simulink model "bh_test_generic_MLFB_model"  (R2021a)
settings: Solver=ode4  StartTime=0.0  StopTime=2  FixedStep=0.001  RelTol=1e-3
settings Model: Creator=bhorton  LastModifiedBy=bhorton
settings DataIOCC: SignalLogging=off  DSMLogging=off  SaveTime=off

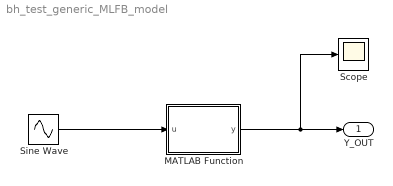
== system bh_test_generic_MLFB_model ==
  MATLAB Function : MATLAB Function  TreatAsAtomicUnit=on
  Scope : Scope
  Sine Wave : Sin  Frequency=2*pi*1  SampleTime=0
  Y_OUT : Outport
  wires:
  Sine Wave/1 -> MATLAB Function/1(u)
  MATLAB Function/1(y) -> Scope/1, Y_OUT/1

== matlab function bh_test_generic_MLFB_model/MATLAB Function ==
  data: u input; y output
function y = fcn(u)

         y = 5*u;

end
